simulink model "FMS"  (R2018b)
settings: configuration reference "fms_config" (kept outside this file)
undefined symbols (not defined in the file): actuator_cmd, ay_cmd, ControlMode, ctrl_mode, DiscIntNeverNeededParam, FMS_Cmd, FMS_CONST, FMS_EXPORT, FMS_PARAM, home, mode, p_cmd, phi_cmd, PilotMode, psi_rate_cmd, q_cmd, r_cmd, reset, state, status, theta_cmd, throttle_cmd, timestamp, u_cmd, v_cmd, VehicleState, VehicleStatus, w_cmd, wp_consume, wp_current
libraries: FMT_Model_Lib x41, simulink x27
(part 2 of 4)

== system FMS/FMS_Commander/Commander/Arm/Assist/Altitude/Heading Command ==
  FMS_In : Inport
  Bus Selector : BusSelector  OutputSignals=Pilot_Cmd.stick_yaw
  DeadZone : Subsystem  mask{th=FMS_PARAM.YAW_DZ}
      mask prompts: th "Threshold"
      mask Display: disp('Dead Zone')
  Gain1 : Gain  Gain=FMS_PARAM.YAW_RATE_LIM  OutDataTypeStr=single
  TD : Subsystem
  psi_rate_cmd_radPs : Outport  VectorParamsAs1DForOutWhenUnconnected=off
  wires:
  FMS_In/1 -> Bus Selector/1
  DeadZone/1(y) -> Gain1/1
  Bus Selector/1 -> DeadZone/1(u)  "<stick_yaw>"
  Gain1/1 -> TD/1(v)
  TD/1(v1) -> psi_rate_cmd_radPs/1

== system FMS/FMS_Commander/Commander/Arm/Assist/Position/Airspeed Command ==
  FMS_In : Inport
  Bias : Bias  Bias=1
  Bus Selector : BusSelector  OutputSignals=Pilot_Cmd.stick_throttle
  Gain : Gain  Gain=FMS_PARAM.FW_AIRSPD_MAX
  Gain1 : Gain  Gain=0.5
  Saturation : Saturate  UpperLimit=1  LowerLimit=0
  u_cmd_mPs : Outport  VectorParamsAs1DForOutWhenUnconnected=off
  wires:
  FMS_In/1 -> Bus Selector/1
  Gain/1 -> u_cmd_mPs/1
  Bus Selector/1 -> Bias/1  "<stick_throttle>"
  Bias/1 -> Gain1/1
  Gain1/1 -> Saturation/1
  Saturation/1 -> Gain/1

== system FMS/FMS_Commander/Commander/Arm/Assist/Position/Altitude Command ==
  FMS_In : Inport
  Controller : Subsystem
  Detect Movement : Subsystem
  w_cmd_mPs : Outport  VectorParamsAs1DForOutWhenUnconnected=off
  wires:
  Controller/1(w_cmd_mPs) -> w_cmd_mPs/1
  Detect Movement/1(motion_state) -> Controller/1(motion_state)
  FMS_In/1 -> Controller/2(FMS_In), Detect Movement/1(FMS_In)

== system FMS/FMS_Commander/Commander/Arm/Assist/Position/Heading Command ==
  FMS_In : Inport
  Bus Selector : BusSelector  OutputSignals=Pilot_Cmd.stick_yaw
  DeadZone : Subsystem  mask{th=FMS_PARAM.YAW_DZ}
      mask prompts: th "Threshold"
      mask Display: disp('Dead Zone')
  Gain1 : Gain  Gain=FMS_PARAM.YAW_RATE_LIM  OutDataTypeStr=single
  TD : Subsystem
  psi_rate_cmd_radPs : Outport  VectorParamsAs1DForOutWhenUnconnected=off
  wires:
  Gain1/1 -> TD/1(v)
  FMS_In/1 -> Bus Selector/1
  DeadZone/1(y) -> Gain1/1
  Bus Selector/1 -> DeadZone/1(u)  "<stick_yaw>"
  TD/1(v1) -> psi_rate_cmd_radPs/1

== system FMS/FMS_Commander/Commander/Arm/Assist/Position/Position Command ==
  FMS_In : Inport
  Controller : Subsystem
  Detect Movement : Subsystem
  ay_cmd_mPs2 : Outport  VectorParamsAs1DForOutWhenUnconnected=off
  wires:
  FMS_In/1 -> Controller/2(FMS_In), Detect Movement/1(FMS_In)
  Controller/1(ay_cmd_mPs2) -> ay_cmd_mPs2/1
  Detect Movement/1(motion_state) -> Controller/1(motion_state)

== system FMS/FMS_Commander/Commander/Arm/Assist/Stabilize/Attitude Command ==
  FMS_In : Inport
  Bus Selector : BusSelector  OutputSignals=Pilot_Cmd.stick_roll,Pilot_Cmd.stick_pitch
  DeadZone : Subsystem  mask{th=FMS_PARAM.ROLL_DZ}
      mask prompts: th "Threshold"
      mask Display: disp('Dead Zone')
  DeadZone2 : Subsystem  mask{th=FMS_PARAM.PITCH_DZ}
      mask prompts: th "Threshold"
      mask Display: disp('Dead Zone')
  Gain : Gain  Gain=FMS_PARAM.ROLL_LIM
  Gain1 : Gain  Gain=-FMS_PARAM.PITCH_LIM
  Phi_CMD_TD : Subsystem  Commented=on
  Theta_CMD_TD : Subsystem  Commented=on
  phi_cmd_radPs : Outport  VectorParamsAs1DForOutWhenUnconnected=off
  theta_cmd_radPs : Outport  Port=2  VectorParamsAs1DForOutWhenUnconnected=off
  wires:
  Bus Selector/2 -> DeadZone2/1(u)  "<stick_pitch>"
  Bus Selector/1 -> DeadZone/1(u)  "<stick_roll>"
  FMS_In/1 -> Bus Selector/1
  DeadZone2/1(y) -> Gain1/1
  DeadZone/1(y) -> Gain/1
  Gain/1 -> phi_cmd_radPs/1
  Gain1/1 -> theta_cmd_radPs/1

== system FMS/FMS_Commander/Commander/Arm/Assist/Stabilize/Heading Command ==
  FMS_In : Inport
  Bus Selector : BusSelector  OutputSignals=Pilot_Cmd.stick_yaw
  DeadZone : Subsystem  mask{th=FMS_PARAM.YAW_DZ}
      mask prompts: th "Threshold"
      mask Display: disp('Dead Zone')
  Gain1 : Gain  Gain=FMS_PARAM.YAW_RATE_LIM  OutDataTypeStr=single
  TD : Subsystem  Commented=on
  psi_rate_cmd_radPs : Outport  VectorParamsAs1DForOutWhenUnconnected=off
  wires:
  Gain1/1 -> psi_rate_cmd_radPs/1
  FMS_In/1 -> Bus Selector/1
  DeadZone/1(y) -> Gain1/1
  Bus Selector/1 -> DeadZone/1(u)  "<stick_yaw>"

== system FMS/FMS_Commander/Commander/Arm/Assist/Stabilize/Throttle Command ==
  FMS_In : Inport
  Add : Sum
  Bus Selector : BusSelector  OutputSignals=Pilot_Cmd.stick_throttle
  Constant4 : Constant  OutDataTypeStr=single
  Constant5 : Constant  Value=1000  OutDataTypeStr=uint16
  Gain2 : Gain  Gain=500  OutDataTypeStr=uint16
  Saturation : Saturate  UpperLimit=2  LowerLimit=0
  Sum : Sum  Inputs=|++
  throttle_cmd : Outport  VectorParamsAs1DForOutWhenUnconnected=off
  wires:
  FMS_In/1 -> Bus Selector/1
  Gain2/1 -> Add/1
  Sum/1 -> Saturation/1
  Saturation/1 -> Gain2/1
  Bus Selector/1 -> Sum/1  "<stick_throttle>"
  Constant5/1 -> Add/2
  Add/1 -> throttle_cmd/1
  Constant4/1 -> Sum/2

== system FMS/FMS_Commander/Commander/Arm/Auto/Mission/Mission_SubSystem ==
  FMS_In : Inport
  Reset : ResetPort  DisableCoverage=on
  Altitude Control : Subsystem
  Bus Assignment : BusAssignment  AssignedSignals=status,state,ctrl_mode,u_cmd,ay_cmd,w_cmd
  Constant : Constant  Value=0  OutDataTypeStr=Bus: FMS_Out_Bus
  Constant1 : Constant  Value=VehicleStatus.Arm
  Constant2 : Constant  Value=VehicleState.Mission
  Constant3 : Constant  Value=ControlMode.POSCTL
  Cruise Speed : Subsystem
  Data Type Conversion : DataTypeConversion
  Data Type Conversion1 : DataTypeConversion
  Data Type Conversion2 : DataTypeConversion
  Position Command : Subsystem
  FMS_Out : Outport  VectorParamsAs1DForOutWhenUnconnected=off
  wires:
  Data Type Conversion1/1 -> Bus Assignment/3
  Constant1/1 -> Data Type Conversion/1
  Data Type Conversion2/1 -> Bus Assignment/4
  Data Type Conversion/1 -> Bus Assignment/2
  Constant2/1 -> Data Type Conversion1/1
  Constant3/1 -> Data Type Conversion2/1
  Constant/1 -> Bus Assignment/1
  Bus Assignment/1 -> FMS_Out/1
  Position Command/1(ay_cmd_mPs2) -> Bus Assignment/6
  Altitude Control/1(w_cmd_mPs) -> Bus Assignment/7
  Cruise Speed/1(cruise_speed) -> Bus Assignment/5
  FMS_In/1 -> Cruise Speed/1(FMS_In), Altitude Control/1(FMS_In), Position Command/1(FMS_In)

== system FMS/FMS_Commander/Commander/Arm/Manual/Manual_Cmd/throttle ==
  stick_throttle : Inport
  Add : Sum
  Constant4 : Constant  OutDataTypeStr=single
  Constant5 : Constant  Value=1000  OutDataTypeStr=single
  Gain4 : Gain  Gain=500  OutDataTypeStr=Inherit: Same as input
  Saturation : Saturate  UpperLimit=2  LowerLimit=0
  Sum : Sum  Inputs=|++
  throttle_cmd : Outport  VectorParamsAs1DForOutWhenUnconnected=off
  wires:
  stick_throttle/1 -> Sum/1
  Sum/1 -> Saturation/1
  Constant4/1 -> Sum/2
  Saturation/1 -> Gain4/1
  Add/1 -> throttle_cmd/1
  Gain4/1 -> Add/1
  Constant5/1 -> Add/2

== system FMS/FMS_Commander/Commander/Arm/SubMode/Hold/Altitude_Hold ==
  FMS_In : Inport
  Bus_Selection : Subsystem
  Delay : Delay  DelayLength=1  InitialConditionSource=Input port
      settings: InputPortMap=u0,p4
  Gain2 : Gain  Gain=FMS_PARAM.Z_P  OutDataTypeStr=single
  Saturation1 : Saturate  UpperLimit=FMS_PARAM.VEL_Z_LIM  LowerLimit=-FMS_PARAM.VEL_Z_LIM
  Sum : Sum  Inputs=-+|
  w_cmd_mPs : Outport  VectorParamsAs1DForOutWhenUnconnected=off
  wires:
  Gain2/1 -> Saturation1/1
  Bus_Selection/1(z_R_m) -> Delay/2, Sum/1  "z_est_R"
  Sum/1 -> Gain2/1  "z_err_R"
  Delay/1 -> Sum/2, Delay/1  "z_cmd_R"
  FMS_In/1 -> Bus_Selection/1(FMS_In)
  Saturation1/1 -> w_cmd_mPs/1

== system FMS/FMS_Commander/Commander/Arm/SubMode/Hold/Loiter_Control ==
  FMS_In : Inport
  Bus Selector2 : BusSelector  OutputSignals=INS_Out.vn,INS_Out.ve
  L1 : Constant  Value=FMS_PARAM.L1  OutDataTypeStr=single
  L1 Reference WP : Subsystem
  L1_Core : Subsystem
  Mux1 : Mux  Inputs=2
  R : Constant  Value=FMS_PARAM.LOITER_R  OutDataTypeStr=single
  Reference_Point : Subsystem
  ay_cmd_mPs2 : Outport  VectorParamsAs1DForOutWhenUnconnected=off
  wires:
  L1 Reference WP/1(L1_WP) -> L1_Core/2(L1_WP)  "L1_WP"
  L1_Core/1(ay_cmd_mPs2) -> ay_cmd_mPs2/1
  Reference_Point/1(p_vehicle) -> L1_Core/1(p_vehicle), L1 Reference WP/1(P_Vehicle)
  Reference_Point/2(p_0) -> L1 Reference WP/2(P_0)
  Reference_Point/3(n) -> L1 Reference WP/3(n)
  R/1 -> L1 Reference WP/4(R)
  L1/1 -> L1_Core/3(L1), L1 Reference WP/5(L1)
  FMS_In/1 -> Bus Selector2/1, Reference_Point/1(FMS_In)
  Bus Selector2/2 -> Mux1/2  "<ve>"
  Bus Selector2/1 -> Mux1/1  "<vn>"
  Mux1/1 -> L1_Core/4(Vg)

== system FMS/FMS_Commander/Commander/Arm/SubMode/Return/Altitude Control ==
  FMS_In : Inport
  Bus Selector3 : BusSelector  OutputSignals=INS_Out.h_R
  Gain : Gain  Gain=FMS_PARAM.Z_P
  Saturation1 : Saturate  UpperLimit=FMS_PARAM.VEL_Z_LIM  LowerLimit=-FMS_PARAM.VEL_Z_LIM
  Sum2 : Sum  Inputs=|+-
  Target Height : Subsystem
  w_cmd_mPs : Outport  VectorParamsAs1DForOutWhenUnconnected=off
  wires:
  FMS_In/1 -> Bus Selector3/1, Target Height/1(FMS_In)
  Bus Selector3/1 -> Sum2/1  "<h_R>"
  Sum2/1 -> Gain/1
  Gain/1 -> Saturation1/1
  Target Height/1(h_R_sp) -> Sum2/2  "h_R_sp"
  Saturation1/1 -> w_cmd_mPs/1

== system FMS/FMS_Commander/Commander/Arm/SubMode/Return/Cruise Speed ==
  FMS_In : Inport
  Bus Selector : BusSelector  OutputSignals=Cmd_In.set_speed
  Compare To Zero : simulink/Logic and Bit Operations/Compare To Zero  relop=>  OutDataTypeStr=boolean
  Switch2 : Switch  Criteria=u2 > Threshold
  vel : Constant  Value=FMS_PARAM.CRUISE_SPEED  OutDataTypeStr=single
  cruise_speed : Outport  VectorParamsAs1DForOutWhenUnconnected=off
  wires:
  Bus Selector/1 -> Compare To Zero/1, Switch2/1  "<set_speed>"
  vel/1 -> Switch2/3  "|Vg|"
  Compare To Zero/1 -> Switch2/2
  Switch2/1 -> cruise_speed/1
  FMS_In/1 -> Bus Selector/1

== system FMS/FMS_Commander/Commander/Arm/SubMode/Return/Position Command ==
  FMS_In : Inport
  L1 Control : Subsystem
  WayPoints : Subsystem
  ay_cmd_mPs2 : Outport  VectorParamsAs1DForOutWhenUnconnected=off
  wires:
  FMS_In/1 -> L1 Control/4(FMS_In), WayPoints/1(FMS_In)
  L1 Control/1(ay_cmd_mPs2) -> ay_cmd_mPs2/1
  WayPoints/2(p2) -> L1 Control/2(p2)
  WayPoints/3(p3) -> L1 Control/3(p3)
  WayPoints/1(p1) -> L1 Control/1(p1)

== system FMS/FMS_Commander/Commander/Arm/SubMode/Takeoff/Altitude Control ==
  FMS_In : Inport
  Bus Selector3 : BusSelector  OutputSignals=INS_Out.h_R
  Gain : Gain  Gain=FMS_PARAM.Z_P
  Saturation1 : Saturate  UpperLimit=FMS_PARAM.VEL_Z_LIM  LowerLimit=-FMS_PARAM.VEL_Z_LIM
  Sum2 : Sum  Inputs=|+-
  Target Height : Subsystem
  w_cmd_mPs : Outport  VectorParamsAs1DForOutWhenUnconnected=off
  wires:
  FMS_In/1 -> Bus Selector3/1, Target Height/1(FMS_In)
  Bus Selector3/1 -> Sum2/1  "<h_R>"
  Sum2/1 -> Gain/1
  Gain/1 -> Saturation1/1
  Target Height/1(h_R_sp) -> Sum2/2  "h_R_sp"
  Saturation1/1 -> w_cmd_mPs/1

== system FMS/FMS_Commander/Commander/Arm/SubMode/Takeoff/Position Command ==
  FMS_In : Inport
  L1 Control : Subsystem
  WayPoints : Subsystem
  ay_cmd_mPs2 : Outport  VectorParamsAs1DForOutWhenUnconnected=off
  wires:
  FMS_In/1 -> L1 Control/4(FMS_In), WayPoints/1(FMS_In)
  L1 Control/1(ay_cmd_mPs2) -> ay_cmd_mPs2/1
  WayPoints/2(p2) -> L1 Control/2(p2)
  WayPoints/3(p3) -> L1 Control/3(p3)
  WayPoints/1(p1) -> L1 Control/1(p1)

== system FMS/FMS_Commander/Commander/Arm/Assist/Altitude/Airspeed Command/TD ==
  v : Inport
  Integrator : DiscreteIntegrator  SampleTime=-1  ICPrevOutput=DiscIntNeverNeededParam  ICPrevScaledInput=DiscIntNeverNeededParam
  Integrator1 : DiscreteIntegrator  SampleTime=-1  ICPrevOutput=DiscIntNeverNeededParam  ICPrevScaledInput=DiscIntNeverNeededParam
  Subtract : Sum  Inputs=+-
  "fhan " : Subsystem  mask{r0=8*9.806, h0=0.05}
      mask DialogControl ParameterGroupVar Prompt: fhan(v1,v2,r0,h0)
  v1 : Outport  VectorParamsAs1DForOutWhenUnconnected=off
  wires:
  Integrator1/1 -> v1/1, Subtract/1
  v/1 -> Subtract/2
  Integrator/1 -> "fhan "/2(v2), Integrator1/1  "v2"
  Subtract/1 -> "fhan "/1(v1)
  "fhan "/1(fhan) -> Integrator/1

== system FMS/FMS_Commander/Commander/Arm/Assist/Altitude/Altitude Command/Controller ==
  motion_state : Inport
  In Bus Element : Inport  Port=2  PortName=FMS_In
  In Bus Element1 : Inport  Port=2  PortName=FMS_In
  Brake Control : Subsystem  TreatAsAtomicUnit=on
  Hold Control : Subsystem  TreatAsAtomicUnit=on
  Merge : Merge  Inputs=3
  Move Control : Subsystem  TreatAsAtomicUnit=on
  Saturation1 : Saturate  UpperLimit=FMS_PARAM.VEL_Z_LIM  LowerLimit=-FMS_PARAM.VEL_Z_LIM
  Switch Case : SwitchCase  CaseConditions={MotionState.Hold, MotionState.Brake, MotionState.Move}  ShowDefaultCase=off
  w_cmd_mPs : Outport  VectorParamsAs1DForOutWhenUnconnected=off
  wires:
  Move Control/1(w_cmd_mPs) -> Merge/3
  Brake Control/1(psi_rate_cmd_radPs) -> Merge/2
  Hold Control/1(w_cmd_mPs) -> Merge/1
  In Bus Element/1 -> Hold Control/1(FMS_In)
  Switch Case/3 -> Move Control/Action
  Switch Case/2 -> Brake Control/Action
  Switch Case/1 -> Hold Control/Action
  motion_state/1 -> Switch Case/1
  Saturation1/1 -> w_cmd_mPs/1
  Merge/1 -> Saturation1/1
  In Bus Element1/1 -> Move Control/1(FMS_In)

== system FMS/FMS_Commander/Commander/Arm/Assist/Altitude/Altitude Command/Detect Movement ==
  FMS_In : Inport
  Abs : Abs
  Abs1 : Abs
  Bus Selector : BusSelector  OutputSignals=Pilot_Cmd.stick_pitch,INS_Out.vd
  Compare To Constant : simulink/Logic and Bit Operations/Compare To Constant  relop=>  const=FMS_PARAM.PITCH_DZ  OutDataTypeStr=boolean
  Motion Status : Stateflow chart  TreatAsAtomicUnit=on
  motion_state : Outport  VectorParamsAs1DForOutWhenUnconnected=off
  wires:
  FMS_In/1 -> Bus Selector/1
  Abs1/1 -> Compare To Constant/1
  Motion Status/1(state) -> motion_state/1
  Compare To Constant/1 -> Motion Status/1(motion_req)
  Abs/1 -> Motion Status/2(speed)
  Bus Selector/1 -> Abs1/1  "<stick_pitch>"
  Bus Selector/2 -> Abs/1  "<vd>"

== system FMS/FMS_Commander/Commander/Arm/Assist/Altitude/Attitude Command/DeadZone ==
  u : Inport
  Dead Zone : DeadZone  LowerValue=-th  UpperValue=th  SaturateOnIntegerOverflow=on
  Gain : Gain  Gain=1/(1-th)
  y : Outport  VectorParamsAs1DForOutWhenUnconnected=off
  wires:
  Gain/1 -> y/1
  Dead Zone/1 -> Gain/1
  u/1 -> Dead Zone/1

== system FMS/FMS_Commander/Commander/Arm/Assist/Altitude/Attitude Command/Phi_CMD_TD ==
  v : Inport
  Integrator : DiscreteIntegrator  SampleTime=-1  ICPrevOutput=DiscIntNeverNeededParam  ICPrevScaledInput=DiscIntNeverNeededParam
  Integrator1 : DiscreteIntegrator  SampleTime=-1  ICPrevOutput=DiscIntNeverNeededParam  ICPrevScaledInput=DiscIntNeverNeededParam
  Subtract : Sum  Inputs=+-
  "fhan " : Subsystem  mask{r0=4*pi, h0=0.04}
      mask DialogControl ParameterGroupVar Prompt: fhan(v1,v2,r0,h0)
  v1 : Outport  VectorParamsAs1DForOutWhenUnconnected=off
  wires:
  "fhan "/1(fhan) -> Integrator/1
  Subtract/1 -> "fhan "/1(v1)
  Integrator/1 -> Integrator1/1, "fhan "/2(v2)  "v2"
  v/1 -> Subtract/2
  Integrator1/1 -> Subtract/1, v1/1

== system FMS/FMS_Commander/Commander/Arm/Assist/Altitude/Heading Command/DeadZone ==
  u : Inport
  Dead Zone : DeadZone  LowerValue=-th  UpperValue=th  SaturateOnIntegerOverflow=on
  Gain : Gain  Gain=1/(1-th)
  y : Outport  VectorParamsAs1DForOutWhenUnconnected=off
  wires:
  Gain/1 -> y/1
  Dead Zone/1 -> Gain/1
  u/1 -> Dead Zone/1

== system FMS/FMS_Commander/Commander/Arm/Assist/Altitude/Heading Command/TD ==
  v : Inport
  Integrator : DiscreteIntegrator  SampleTime=-1  ICPrevOutput=DiscIntNeverNeededParam  ICPrevScaledInput=DiscIntNeverNeededParam
  Integrator1 : DiscreteIntegrator  SampleTime=-1  ICPrevOutput=DiscIntNeverNeededParam  ICPrevScaledInput=DiscIntNeverNeededParam
  Subtract : Sum  Inputs=+-
  "fhan " : Subsystem  mask{r0=5*pi, h0=0.02}
      mask DialogControl ParameterGroupVar Prompt: fhan(v1,v2,r0,h0)
  v1 : Outport  VectorParamsAs1DForOutWhenUnconnected=off
  wires:
  "fhan "/1(fhan) -> Integrator/1
  Subtract/1 -> "fhan "/1(v1)
  Integrator/1 -> Integrator1/1, "fhan "/2(v2)  "v2"
  v/1 -> Subtract/2
  Integrator1/1 -> Subtract/1, v1/1

== system FMS/FMS_Commander/Commander/Arm/Assist/Position/Altitude Command/Controller ==
  motion_state : Inport
  In Bus Element : Inport  Port=2  PortName=FMS_In
  In Bus Element1 : Inport  Port=2  PortName=FMS_In
  Brake Control : Subsystem  TreatAsAtomicUnit=on
  Hold Control : Subsystem  TreatAsAtomicUnit=on
  Merge : Merge  Inputs=3
  Move Control : Subsystem  TreatAsAtomicUnit=on
  Saturation1 : Saturate  UpperLimit=FMS_PARAM.VEL_Z_LIM  LowerLimit=-FMS_PARAM.VEL_Z_LIM
  Switch Case : SwitchCase  CaseConditions={MotionState.Hold, MotionState.Brake, MotionState.Move}  ShowDefaultCase=off
  w_cmd_mPs : Outport  VectorParamsAs1DForOutWhenUnconnected=off
  wires:
  Move Control/1(w_cmd_mPs) -> Merge/3
  Brake Control/1(psi_rate_cmd_radPs) -> Merge/2
  Hold Control/1(w_cmd_mPs) -> Merge/1
  In Bus Element/1 -> Hold Control/1(FMS_In)
  Switch Case/3 -> Move Control/Action
  Switch Case/2 -> Brake Control/Action
  Switch Case/1 -> Hold Control/Action
  motion_state/1 -> Switch Case/1
  Saturation1/1 -> w_cmd_mPs/1
  Merge/1 -> Saturation1/1
  In Bus Element1/1 -> Move Control/1(FMS_In)

== system FMS/FMS_Commander/Commander/Arm/Assist/Position/Altitude Command/Detect Movement ==
  FMS_In : Inport
  Abs : Abs
  Abs1 : Abs
  Bus Selector : BusSelector  OutputSignals=Pilot_Cmd.stick_pitch,INS_Out.vd
  Compare To Constant : simulink/Logic and Bit Operations/Compare To Constant  relop=>  const=FMS_PARAM.PITCH_DZ  OutDataTypeStr=boolean
  Motion Status : Stateflow chart  TreatAsAtomicUnit=on
  motion_state : Outport  VectorParamsAs1DForOutWhenUnconnected=off
  wires:
  FMS_In/1 -> Bus Selector/1
  Abs1/1 -> Compare To Constant/1
  Motion Status/1(state) -> motion_state/1
  Compare To Constant/1 -> Motion Status/1(motion_req)
  Abs/1 -> Motion Status/2(speed)
  Bus Selector/1 -> Abs1/1  "<stick_pitch>"
  Bus Selector/2 -> Abs/1  "<vd>"

== system FMS/FMS_Commander/Commander/Arm/Assist/Position/Heading Command/DeadZone ==
  u : Inport
  Dead Zone : DeadZone  LowerValue=-th  UpperValue=th  SaturateOnIntegerOverflow=on
  Gain : Gain  Gain=1/(1-th)
  y : Outport  VectorParamsAs1DForOutWhenUnconnected=off
  wires:
  Gain/1 -> y/1
  Dead Zone/1 -> Gain/1
  u/1 -> Dead Zone/1

== system FMS/FMS_Commander/Commander/Arm/Assist/Position/Heading Command/TD ==
  v : Inport
  Integrator : DiscreteIntegrator  SampleTime=-1  ICPrevOutput=DiscIntNeverNeededParam  ICPrevScaledInput=DiscIntNeverNeededParam
  Integrator1 : DiscreteIntegrator  SampleTime=-1  ICPrevOutput=DiscIntNeverNeededParam  ICPrevScaledInput=DiscIntNeverNeededParam
  Subtract : Sum  Inputs=+-
  "fhan " : Subsystem  mask{r0=5*pi, h0=0.02}
      mask DialogControl ParameterGroupVar Prompt: fhan(v1,v2,r0,h0)
  v1 : Outport  VectorParamsAs1DForOutWhenUnconnected=off
  wires:
  "fhan "/1(fhan) -> Integrator/1
  Subtract/1 -> "fhan "/1(v1)
  Integrator/1 -> Integrator1/1, "fhan "/2(v2)  "v2"
  v/1 -> Subtract/2
  Integrator1/1 -> Subtract/1, v1/1

== system FMS/FMS_Commander/Commander/Arm/Assist/Position/Position Command/Controller ==
  motion_state : Inport
  In Bus Element : Inport  Port=2  PortName=FMS_In
  In Bus Element1 : Inport  Port=2  PortName=FMS_In
  Brake Control : Subsystem  TreatAsAtomicUnit=on
  Hold Control : Subsystem  TreatAsAtomicUnit=on
  Merge : Merge  Inputs=3
  Move Control : Subsystem  TreatAsAtomicUnit=on
  Saturation1 : Saturate  UpperLimit=FMS_PARAM.ACC_Y_LIM  LowerLimit=-FMS_PARAM.ACC_Y_LIM
  Switch Case : SwitchCase  CaseConditions={MotionState.Hold, MotionState.Brake, MotionState.Move}  ShowDefaultCase=off
  ay_cmd_mPs2 : Outport  VectorParamsAs1DForOutWhenUnconnected=off
  wires:
  Move Control/1(ay_cmd_mPs2) -> Merge/3
  Brake Control/1(ay_cmd_mPs2) -> Merge/2
  Hold Control/1(ay_cmd_mPs2) -> Merge/1
  In Bus Element/1 -> Hold Control/1(FMS_In)
  Switch Case/3 -> Move Control/Action
  Switch Case/2 -> Brake Control/Action
  Switch Case/1 -> Hold Control/Action
  motion_state/1 -> Switch Case/1
  Saturation1/1 -> ay_cmd_mPs2/1
  Merge/1 -> Saturation1/1
  In Bus Element1/1 -> Move Control/1(FMS_In)

== system FMS/FMS_Commander/Commander/Arm/Assist/Position/Position Command/Detect Movement ==
  FMS_In : Inport
  Abs : Abs
  Abs1 : Abs
  Bus Selector1 : BusSelector  OutputSignals=Pilot_Cmd.stick_roll
  Bus Selector2 : BusSelector  OutputSignals=INS_Out.psi,INS_Out.vn,INS_Out.ve,INS_Out.vd
  Compare To Constant : simulink/Logic and Bit Operations/Compare To Constant  relop=>  const=FMS_PARAM.ROLL_DZ  OutDataTypeStr=boolean
  Motion State : Stateflow chart  TreatAsAtomicUnit=on
  Multiply : Product  Multiplication=Matrix(*)
  Mux : Mux  Inputs=3
  Psi To DCM : FMT_Model_Lib/Transformation/Psi To DCM
      settings: SourceProductName=FMT Toolbox
  Selector : Selector  InputPortWidth=3  IndexOptions=Index vector (dialog)  Indices=2  OutputSizes=1
  motion_state : Outport  VectorParamsAs1DForOutWhenUnconnected=off
  wires:
  FMS_In/1 -> Bus Selector2/1, Bus Selector1/1
  Compare To Constant/1 -> Motion State/1(motion_req)
  Abs1/1 -> Compare To Constant/1
  Motion State/1(state) -> motion_state/1  "pos_ms"
  Abs/1 -> Motion State/2(speed)
  Bus Selector1/1 -> Abs1/1  "<stick_roll>"
  Bus Selector2/1 -> Psi To DCM/1  "<psi>"
  Bus Selector2/2 -> Mux/1  "<vn>"
  Bus Selector2/3 -> Mux/2  "<ve>"
  Bus Selector2/4 -> Mux/3  "<vd>"
  Psi To DCM/1 -> Multiply/1
  Multiply/1 -> Selector/1
  Selector/1 -> Abs/1
  Mux/1 -> Multiply/2

== system FMS/FMS_Commander/Commander/Arm/Assist/Stabilize/Attitude Command/DeadZone ==
  u : Inport
  Dead Zone : DeadZone  LowerValue=-th  UpperValue=th  SaturateOnIntegerOverflow=on
  Gain : Gain  Gain=1/(1-th)
  y : Outport  VectorParamsAs1DForOutWhenUnconnected=off
  wires:
  Gain/1 -> y/1
  Dead Zone/1 -> Gain/1
  u/1 -> Dead Zone/1

== system FMS/FMS_Commander/Commander/Arm/Assist/Stabilize/Attitude Command/DeadZone2 ==
  u : Inport
  Dead Zone : DeadZone  LowerValue=-th  UpperValue=th  SaturateOnIntegerOverflow=on
  Gain : Gain  Gain=1/(1-th)
  y : Outport  VectorParamsAs1DForOutWhenUnconnected=off
  wires:
  u/1 -> Dead Zone/1
  Dead Zone/1 -> Gain/1
  Gain/1 -> y/1

== system FMS/FMS_Commander/Commander/Arm/Assist/Stabilize/Attitude Command/Phi_CMD_TD ==
  v : Inport
  Integrator : DiscreteIntegrator  SampleTime=-1  ICPrevOutput=DiscIntNeverNeededParam  ICPrevScaledInput=DiscIntNeverNeededParam
  Integrator1 : DiscreteIntegrator  SampleTime=-1  ICPrevOutput=DiscIntNeverNeededParam  ICPrevScaledInput=DiscIntNeverNeededParam
  Subtract : Sum  Inputs=+-
  "fhan " : Subsystem  mask{r0=4*pi, h0=0.04}
      mask DialogControl ParameterGroupVar Prompt: fhan(v1,v2,r0,h0)
  v1 : Outport  VectorParamsAs1DForOutWhenUnconnected=off
  wires:
  "fhan "/1(fhan) -> Integrator/1
  Subtract/1 -> "fhan "/1(v1)
  Integrator/1 -> Integrator1/1, "fhan "/2(v2)  "v2"
  v/1 -> Subtract/2
  Integrator1/1 -> Subtract/1, v1/1

== system FMS/FMS_Commander/Commander/Arm/Assist/Stabilize/Attitude Command/Theta_CMD_TD ==
  v : Inport
  Integrator : DiscreteIntegrator  SampleTime=-1  ICPrevOutput=DiscIntNeverNeededParam  ICPrevScaledInput=DiscIntNeverNeededParam
  Integrator1 : DiscreteIntegrator  SampleTime=-1  ICPrevOutput=DiscIntNeverNeededParam  ICPrevScaledInput=DiscIntNeverNeededParam
  Subtract : Sum  Inputs=+-
  "fhan " : Subsystem  mask{r0=4*pi, h0=0.04}
      mask DialogControl ParameterGroupVar Prompt: fhan(v1,v2,r0,h0)
  v1 : Outport  VectorParamsAs1DForOutWhenUnconnected=off
  wires:
  Integrator1/1 -> v1/1, Subtract/1
  v/1 -> Subtract/2
  Integrator/1 -> Integrator1/1, "fhan "/2(v2)  "v2"
  Subtract/1 -> "fhan "/1(v1)
  "fhan "/1(fhan) -> Integrator/1

== system FMS/FMS_Commander/Commander/Arm/Assist/Stabilize/Heading Command/DeadZone ==
  u : Inport
  Dead Zone : DeadZone  LowerValue=-th  UpperValue=th  SaturateOnIntegerOverflow=on
  Gain : Gain  Gain=1/(1-th)
  y : Outport  VectorParamsAs1DForOutWhenUnconnected=off
  wires:
  Gain/1 -> y/1
  Dead Zone/1 -> Gain/1
  u/1 -> Dead Zone/1

== system FMS/FMS_Commander/Commander/Arm/Assist/Stabilize/Heading Command/TD ==
  v : Inport
  Integrator : DiscreteIntegrator  SampleTime=-1  ICPrevOutput=DiscIntNeverNeededParam  ICPrevScaledInput=DiscIntNeverNeededParam
  Integrator1 : DiscreteIntegrator  SampleTime=-1  ICPrevOutput=DiscIntNeverNeededParam  ICPrevScaledInput=DiscIntNeverNeededParam
  Subtract : Sum  Inputs=+-
  "fhan " : Subsystem  mask{r0=5*pi, h0=0.02}
      mask DialogControl ParameterGroupVar Prompt: fhan(v1,v2,r0,h0)
  v1 : Outport  VectorParamsAs1DForOutWhenUnconnected=off
  wires:
  "fhan "/1(fhan) -> Integrator/1
  Subtract/1 -> "fhan "/1(v1)
  Integrator/1 -> Integrator1/1, "fhan "/2(v2)  "v2"
  v/1 -> Subtract/2
  Integrator1/1 -> Subtract/1, v1/1

== system FMS/FMS_Commander/Commander/Arm/Auto/Mission/Mission_SubSystem/Altitude Control ==
  FMS_In : Inport
  Bus Selector3 : BusSelector  OutputSignals=INS_Out.h_R
  Gain : Gain  Gain=FMS_PARAM.Z_P
  Saturation1 : Saturate  UpperLimit=FMS_PARAM.VEL_Z_LIM  LowerLimit=-FMS_PARAM.VEL_Z_LIM
  Sum2 : Sum  Inputs=|+-
  Target Height : Subsystem
  w_cmd_mPs : Outport  VectorParamsAs1DForOutWhenUnconnected=off
  wires:
  FMS_In/1 -> Bus Selector3/1, Target Height/1(FMS_In)
  Bus Selector3/1 -> Sum2/1  "<h_R>"
  Sum2/1 -> Gain/1
  Gain/1 -> Saturation1/1
  Target Height/1(h_R_sp) -> Sum2/2  "h_R_sp"
  Saturation1/1 -> w_cmd_mPs/1

== system FMS/FMS_Commander/Commander/Arm/Auto/Mission/Mission_SubSystem/Cruise Speed ==
  FMS_In : Inport
  Bus Selector : BusSelector  OutputSignals=Cmd_In.set_speed
  Compare To Zero : simulink/Logic and Bit Operations/Compare To Zero  relop=>  OutDataTypeStr=boolean
  Switch2 : Switch  Criteria=u2 > Threshold
  vel : Constant  Value=FMS_PARAM.CRUISE_SPEED  OutDataTypeStr=single
  cruise_speed : Outport  VectorParamsAs1DForOutWhenUnconnected=off
  wires:
  Bus Selector/1 -> Compare To Zero/1, Switch2/1  "<set_speed>"
  vel/1 -> Switch2/3  "|Vg|"
  Compare To Zero/1 -> Switch2/2
  Switch2/1 -> cruise_speed/1
  FMS_In/1 -> Bus Selector/1

== system FMS/FMS_Commander/Commander/Arm/Auto/Mission/Mission_SubSystem/Position Command ==
  FMS_In : Inport
  L1 Control : Subsystem
  WayPoints : Subsystem
  ay_cmd_mPs2 : Outport  VectorParamsAs1DForOutWhenUnconnected=off
  wires:
  FMS_In/1 -> L1 Control/4(FMS_In), WayPoints/1(FMS_In)
  L1 Control/1(ay_cmd_mPs2) -> ay_cmd_mPs2/1
  WayPoints/2(p2) -> L1 Control/2(p2)
  WayPoints/3(p3) -> L1 Control/3(p3)
  WayPoints/1(p1) -> L1 Control/1(p1)

== system FMS/FMS_Commander/Commander/Arm/SubMode/Hold/Altitude_Hold/Bus_Selection ==
  FMS_In : Inport
  Bus Selector2 : BusSelector  OutputSignals=INS_Out.h_R
  Gain : Gain  Gain=-1
  z_R_m : Outport  VectorParamsAs1DForOutWhenUnconnected=off
  wires:
  Gain/1 -> z_R_m/1
  Bus Selector2/1 -> Gain/1  "<h_R>"
  FMS_In/1 -> Bus Selector2/1

== system FMS/FMS_Commander/Commander/Arm/SubMode/Hold/Loiter_Control/L1 Reference WP ==
  P_Vehicle : Inport
  P_0 : Inport  Port=2
  n : Inport  Port=3
  R : Inport  Port=4
  L1 : Inport  Port=5
  Compare To Constant : simulink/Logic and Bit Operations/Compare To Constant  relop=>  const=0  OutDataTypeStr=boolean
  Gain : Gain  Gain=0.5
  Max : MinMax  Function=max  Inputs=2
  OutRegionRegWP : MATLAB Function  TreatAsAtomicUnit=on
  Reshape : Reshape  OutputDimensionality=Customize  OutputDimensions=[2,1]
  Reshape1 : Reshape  OutputDimensionality=Column vector (2-D)
  Reshape2 : Reshape  OutputDimensionality=Column vector (2-D)
  Reshape3 : Reshape  OutputDimensionality=Column vector (2-D)
  SearchL1RefWP : MATLAB Function  TreatAsAtomicUnit=on
  Switch : Switch  Criteria=u2 > Threshold
  L1_WP : Outport  VectorParamsAs1DForOutWhenUnconnected=off
  wires:
  Reshape/1 -> L1_WP/1
  Compare To Constant/1 -> Switch/2
  SearchL1RefWP/2(n) -> Compare To Constant/1
  OutRegionRegWP/1(P) -> Switch/3
  Switch/1 -> Reshape/1
  SearchL1RefWP/1(P) -> Switch/1
  P_0/1 -> Reshape1/1
  P_Vehicle/1 -> Reshape2/1
  Max/1 -> OutRegionRegWP/3(R), SearchL1RefWP/3(R)
  L1/1 -> Gain/1, OutRegionRegWP/4(L1), SearchL1RefWP/4(L1)
  Reshape1/1 -> OutRegionRegWP/1(P0), SearchL1RefWP/1(P_0)
  Reshape2/1 -> OutRegionRegWP/2(P_Vehicle), SearchL1RefWP/2(P_Vehicle)
  n/1 -> Reshape3/1
  Reshape3/1 -> OutRegionRegWP/5(n)
  R/1 -> Max/1
  Gain/1 -> Max/2

== system FMS/FMS_Commander/Commander/Arm/SubMode/Hold/Loiter_Control/L1_Core ==
  p_vehicle : Inport
  L1_WP : Inport  Port=2
  L1 : Inport  Port=3
  Vg : Inport  Port=4
  L1_Lateral_Acceleration : Subsystem
  Saturation : Saturate  UpperLimit=9.81  LowerLimit=-9.81
  Subtract : Sum  Inputs=+-
  ay_cmd_mPs2 : Outport  VectorParamsAs1DForOutWhenUnconnected=off
  wires:
  L1_WP/1 -> Subtract/1
  p_vehicle/1 -> Subtract/2
  L1/1 -> L1_Lateral_Acceleration/1(L1)
  Vg/1 -> L1_Lateral_Acceleration/2(Vg)
  Subtract/1 -> L1_Lateral_Acceleration/3(l1_path)
  L1_Lateral_Acceleration/1(l1_a_cmd) -> Saturation/1
  Saturation/1 -> ay_cmd_mPs2/1

== system FMS/FMS_Commander/Commander/Arm/SubMode/Hold/Loiter_Control/Reference_Point ==
  FMS_In : Inport
  Bus Selector1 : BusSelector  OutputSignals=Cmd_In.cur_waypoint
  Bus Selector2 : BusSelector  OutputSignals=INS_Out.vn,INS_Out.ve
  Bus Selector3 : BusSelector  OutputSignals=INS_Out.x_R,INS_Out.y_R
  Mux1 : Mux  Inputs=2
  Mux2 : Mux  Inputs=2
  Selector : Selector  InputPortWidth=3  IndexOptions=Index vector (dialog)  Indices=[1 2]  OutputSizes=1
  Vector Normalize : FMT_Model_Lib/Math/Vector Normalize
      settings: SourceProductName=FMT Toolbox
  start_vel : Delay  DelayLength=1  InitialConditionSource=Input port
      settings: InputPortMap=u0,p4
  p_vehicle : Outport  VectorParamsAs1DForOutWhenUnconnected=off
  p_0 : Outport  Port=2  VectorParamsAs1DForOutWhenUnconnected=off
  n : Outport  Port=3  VectorParamsAs1DForOutWhenUnconnected=off
  wires:
  Bus Selector2/2 -> Mux1/2  "<ve>"
  start_vel/1 -> Vector Normalize/1, start_vel/1
  Bus Selector2/1 -> Mux1/1  "<vn>"
  Vector Normalize/1 -> n/1
  FMS_In/1 -> Bus Selector3/1, Bus Selector2/1, Bus Selector1/1
  Mux1/1 -> start_vel/2
  Bus Selector3/1 -> Mux2/1  "<x_R>"
  Bus Selector3/2 -> Mux2/2  "<y_R>"
  Mux2/1 -> p_vehicle/1
  Bus Selector1/1 -> Selector/1  "<cur_waypoint>"
  Selector/1 -> p_0/1

== system FMS/FMS_Commander/Commander/Arm/SubMode/Return/Altitude Control/Target Height ==
  FMS_In : Inport
  Add : Sum
  Bus Selector : BusSelector  OutputSignals=Cmd_In.sp_waypoint,Cmd_In.cur_waypoint
  Bus Selector1 : BusSelector  OutputSignals=INS_Out.x_R,INS_Out.y_R
  Bus Selector2 : BusSelector  OutputSignals=Cmd_In.cur_waypoint,Cmd_In.sp_waypoint
  Divide : Product  Inputs=*/
  Multiply : Product
  Mux : Mux  Inputs=2
  Saturation : Saturate  UpperLimit=1  LowerLimit=0
  Selector : Selector  InputPortWidth=3  IndexOptions=Index vector (dialog)  Indices=3  OutputSizes=1
  Selector1 : Selector  InputPortWidth=3  IndexOptions=Index vector (dialog)  Indices=3  OutputSizes=1
  Selector2 : Selector  InputPortWidth=3  IndexOptions=Index vector (dialog)  Indices=[1 2]  OutputSizes=1
  Selector3 : Selector  InputPortWidth=3  IndexOptions=Index vector (dialog)  Indices=[1 2]  OutputSizes=1
  Subtract : Sum  Inputs=+-
  Sum : Sum  Inputs=|+-
  Sum1 : Sum  Inputs=-+|
  Vector Modulus : FMT_Model_Lib/Math/Vector Modulus
      settings: SourceProductName=FMT Toolbox
  Vector Modulus1 : FMT_Model_Lib/Math/Vector Modulus
      settings: SourceProductName=FMT Toolbox
  h_R_sp : Outport  VectorParamsAs1DForOutWhenUnconnected=off
  wires:
  Multiply/1 -> Add/2
  Bus Selector1/1 -> Mux/1  "<x_R>"
  Bus Selector/1 -> Selector1/1  "<sp_waypoint>"
  Vector Modulus1/1 -> Divide/2
  Sum1/1 -> Vector Modulus1/1
  Sum/1 -> Vector Modulus/1
  Selector2/1 -> Sum1/1, Sum/2
  FMS_In/1 -> Bus Selector2/1, Bus Selector1/1, Bus Selector/1
  Bus Selector2/2 -> Selector3/1  "<sp_waypoint>"
  Vector Modulus/1 -> Divide/1
  Bus Selector1/2 -> Mux/2  "<y_R>"
  Bus Selector2/1 -> Selector2/1  "<cur_waypoint>"
  Selector1/1 -> Subtract/1
  Mux/1 -> Sum/1
  Subtract/1 -> Multiply/1
  Divide/1 -> Saturation/1
  Selector3/1 -> Sum1/2
  Bus Selector/2 -> Selector/1  "<cur_waypoint>"
  Selector/1 -> Add/1, Subtract/2
  Saturation/1 -> Multiply/2
  Add/1 -> h_R_sp/1

== system FMS/FMS_Commander/Commander/Arm/SubMode/Return/Position Command/L1 Control ==
  p1 : Inport
  p2 : Inport  Port=2
  p3 : Inport  Port=3
  FMS_In : Inport  Port=4
  Bus Selector1 : BusSelector  OutputSignals=INS_Out.vn,INS_Out.ve
  L1 : Constant  Value=FMS_PARAM.L1  OutDataTypeStr=single
  L1 Reference WP : Subsystem
  L1_Core : Subsystem
  Mux : Mux  Inputs=2
  Saturation1 : Saturate  UpperLimit=FMS_PARAM.ACC_Y_LIM  LowerLimit=-FMS_PARAM.ACC_Y_LIM
  ay_cmd_mPs2 : Outport  VectorParamsAs1DForOutWhenUnconnected=off
  wires:
  p3/1 -> L1_Core/1(p_vehicle), L1 Reference WP/3(P3)
  p2/1 -> L1 Reference WP/2(P2)
  p1/1 -> L1 Reference WP/1(P1)
  L1/1 -> L1_Core/3(L1), L1 Reference WP/4(L1)
  L1 Reference WP/1(L1_WP) -> L1_Core/2(L1_WP)  "L1_WP"
  Mux/1 -> L1_Core/4(Vg)
  Bus Selector1/1 -> Mux/1  "<vn>"
  Bus Selector1/2 -> Mux/2  "<ve>"
  FMS_In/1 -> Bus Selector1/1
  L1_Core/1(ay_cmd_mPs2) -> Saturation1/1
  Saturation1/1 -> ay_cmd_mPs2/1

== system FMS/FMS_Commander/Commander/Arm/SubMode/Return/Position Command/WayPoints ==
  note: P1: path start point
      | P2: path end point
      | P3: vehicle point
  FMS_In : Inport
  Bus Selector : BusSelector  OutputSignals=INS_Out.x_R,INS_Out.y_R
  Bus Selector1 : BusSelector  OutputSignals=Cmd_In.sp_waypoint
  Bus Selector2 : BusSelector  OutputSignals=Cmd_In.cur_waypoint
  Mux : Mux  Inputs=2
  Reshape : Reshape  OutputDimensionality=Customize  OutputDimensions=[2,1]
  Reshape1 : Reshape  OutputDimensionality=Customize  OutputDimensions=[2,1]
  Reshape2 : Reshape  OutputDimensionality=Customize  OutputDimensions=[2,1]
  Selector : Selector  InputPortWidth=3  IndexOptions=Index vector (dialog)  Indices=[1 2]  OutputSizes=1
  Selector1 : Selector  InputPortWidth=3  IndexOptions=Index vector (dialog)  Indices=[1 2]  OutputSizes=1
  p1 : Outport  VectorParamsAs1DForOutWhenUnconnected=off
  p2 : Outport  Port=2  VectorParamsAs1DForOutWhenUnconnected=off
  p3 : Outport  Port=3  VectorParamsAs1DForOutWhenUnconnected=off
  wires:
  Reshape2/1 -> p3/1
  Reshape1/1 -> p1/1
  Reshape/1 -> p2/1
  Bus Selector/2 -> Mux/2  "<y_R>"
  Bus Selector/1 -> Mux/1  "<x_R>"
  Mux/1 -> Reshape2/1
  Bus Selector1/1 -> Selector/1  "<sp_waypoint>"
  Selector/1 -> Reshape/1
  Selector1/1 -> Reshape1/1
  Bus Selector2/1 -> Selector1/1  "<cur_waypoint>"
  FMS_In/1 -> Bus Selector2/1, Bus Selector1/1, Bus Selector/1

== system FMS/FMS_Commander/Commander/Arm/SubMode/Takeoff/Altitude Control/Target Height ==
  FMS_In : Inport
  Add : Sum
  Bus Selector : BusSelector  OutputSignals=Cmd_In.sp_waypoint,Cmd_In.cur_waypoint
  Bus Selector1 : BusSelector  OutputSignals=INS_Out.x_R,INS_Out.y_R
  Bus Selector2 : BusSelector  OutputSignals=Cmd_In.cur_waypoint,Cmd_In.sp_waypoint
  Divide : Product  Inputs=*/
  Multiply : Product
  Mux : Mux  Inputs=2
  Saturation : Saturate  UpperLimit=1  LowerLimit=0
  Selector : Selector  InputPortWidth=3  IndexOptions=Index vector (dialog)  Indices=3  OutputSizes=1
  Selector1 : Selector  InputPortWidth=3  IndexOptions=Index vector (dialog)  Indices=3  OutputSizes=1
  Selector2 : Selector  InputPortWidth=3  IndexOptions=Index vector (dialog)  Indices=[1 2]  OutputSizes=1
  Selector3 : Selector  InputPortWidth=3  IndexOptions=Index vector (dialog)  Indices=[1 2]  OutputSizes=1
  Subtract : Sum  Inputs=+-
  Sum : Sum  Inputs=|+-
  Sum1 : Sum  Inputs=-+|
  Vector Modulus : FMT_Model_Lib/Math/Vector Modulus
      settings: SourceProductName=FMT Toolbox
  Vector Modulus1 : FMT_Model_Lib/Math/Vector Modulus
      settings: SourceProductName=FMT Toolbox
  h_R_sp : Outport  VectorParamsAs1DForOutWhenUnconnected=off
  wires:
  Multiply/1 -> Add/2
  Bus Selector1/1 -> Mux/1  "<x_R>"
  Bus Selector/1 -> Selector1/1  "<sp_waypoint>"
  Vector Modulus1/1 -> Divide/2
  Sum1/1 -> Vector Modulus1/1
  Sum/1 -> Vector Modulus/1
  Selector2/1 -> Sum1/1, Sum/2
  FMS_In/1 -> Bus Selector2/1, Bus Selector1/1, Bus Selector/1
  Bus Selector2/2 -> Selector3/1  "<sp_waypoint>"
  Vector Modulus/1 -> Divide/1
  Bus Selector1/2 -> Mux/2  "<y_R>"
  Bus Selector2/1 -> Selector2/1  "<cur_waypoint>"
  Selector1/1 -> Subtract/1
  Mux/1 -> Sum/1
  Subtract/1 -> Multiply/1
  Divide/1 -> Saturation/1
  Selector3/1 -> Sum1/2
  Bus Selector/2 -> Selector/1  "<cur_waypoint>"
  Selector/1 -> Add/1, Subtract/2
  Saturation/1 -> Multiply/2
  Add/1 -> h_R_sp/1

== system FMS/FMS_Commander/Commander/Arm/SubMode/Takeoff/Position Command/L1 Control ==
  p1 : Inport
  p2 : Inport  Port=2
  p3 : Inport  Port=3
  FMS_In : Inport  Port=4
  Bus Selector1 : BusSelector  OutputSignals=INS_Out.vn,INS_Out.ve
  L1 : Constant  Value=FMS_PARAM.L1  OutDataTypeStr=single
  L1 Reference WP : Subsystem
  L1_Core : Subsystem
  Mux : Mux  Inputs=2
  Saturation1 : Saturate  UpperLimit=FMS_PARAM.ACC_Y_LIM  LowerLimit=-FMS_PARAM.ACC_Y_LIM
  ay_cmd_mPs2 : Outport  VectorParamsAs1DForOutWhenUnconnected=off
  wires:
  p3/1 -> L1_Core/1(p_vehicle), L1 Reference WP/3(P3)
  p2/1 -> L1 Reference WP/2(P2)
  p1/1 -> L1 Reference WP/1(P1)
  L1/1 -> L1_Core/3(L1), L1 Reference WP/4(L1)
  L1 Reference WP/1(L1_WP) -> L1_Core/2(L1_WP)  "L1_WP"
  Mux/1 -> L1_Core/4(Vg)
  Bus Selector1/1 -> Mux/1  "<vn>"
  Bus Selector1/2 -> Mux/2  "<ve>"
  FMS_In/1 -> Bus Selector1/1
  L1_Core/1(ay_cmd_mPs2) -> Saturation1/1
  Saturation1/1 -> ay_cmd_mPs2/1

== system FMS/FMS_Commander/Commander/Arm/SubMode/Takeoff/Position Command/WayPoints ==
  note: P1: path start point
      | P2: path end point
      | P3: vehicle point
  FMS_In : Inport
  Bus Selector : BusSelector  OutputSignals=INS_Out.x_R,INS_Out.y_R
  Bus Selector1 : BusSelector  OutputSignals=Cmd_In.sp_waypoint
  Bus Selector2 : BusSelector  OutputSignals=Cmd_In.cur_waypoint
  Mux : Mux  Inputs=2
  Reshape : Reshape  OutputDimensionality=Customize  OutputDimensions=[2,1]
  Reshape1 : Reshape  OutputDimensionality=Customize  OutputDimensions=[2,1]
  Reshape2 : Reshape  OutputDimensionality=Customize  OutputDimensions=[2,1]
  Selector : Selector  InputPortWidth=3  IndexOptions=Index vector (dialog)  Indices=[1 2]  OutputSizes=1
  Selector1 : Selector  InputPortWidth=3  IndexOptions=Index vector (dialog)  Indices=[1 2]  OutputSizes=1
  p1 : Outport  VectorParamsAs1DForOutWhenUnconnected=off
  p2 : Outport  Port=2  VectorParamsAs1DForOutWhenUnconnected=off
  p3 : Outport  Port=3  VectorParamsAs1DForOutWhenUnconnected=off
  wires:
  Reshape2/1 -> p3/1
  Reshape1/1 -> p1/1
  Reshape/1 -> p2/1
  Bus Selector/2 -> Mux/2  "<y_R>"
  Bus Selector/1 -> Mux/1  "<x_R>"
  Mux/1 -> Reshape2/1
  FMS_In/1 -> Bus Selector2/1, Bus Selector1/1, Bus Selector/1
  Bus Selector1/1 -> Selector/1  "<sp_waypoint>"
  Selector/1 -> Reshape/1
  Bus Selector2/1 -> Selector1/1  "<cur_waypoint>"
  Selector1/1 -> Reshape1/1

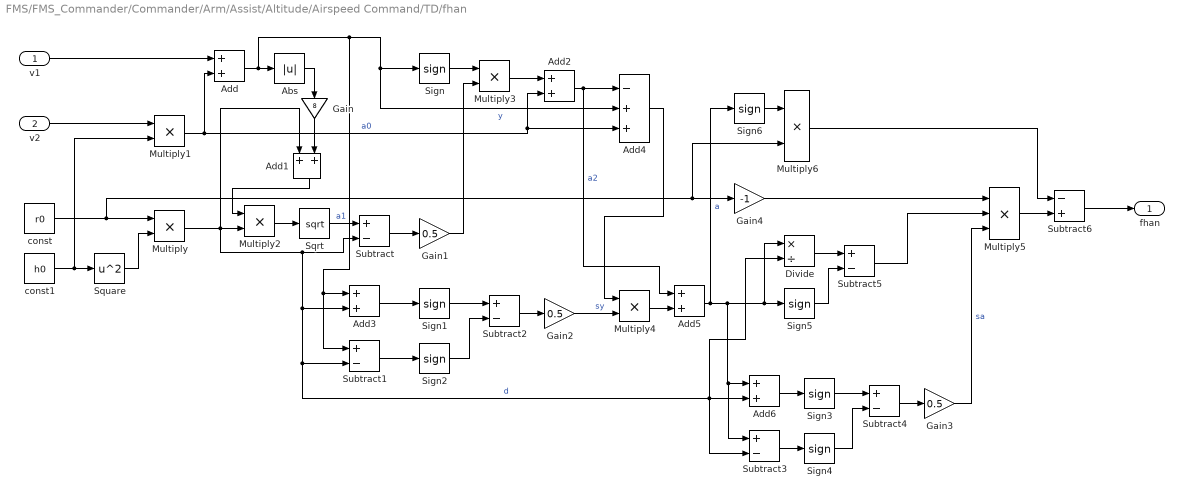
== system FMS/FMS_Commander/Commander/Arm/Assist/Altitude/Airspeed Command/TD/fhan  ==
  v1 : Inport
  v2 : Inport  Port=2
  Abs : Abs
  Add{,1..3,5..6} (6 alike) : Sum  OutDataTypeStr=Inherit: Same as first input
  Add4 : Sum  Inputs=-++
  Divide : Product  Inputs=*/
  Gain : Gain  Gain=8
  Gain1 : Gain  Gain=0.5  OutDataTypeStr=Inherit: Same as input
  Gain2 : Gain  Gain=0.5  OutDataTypeStr=Inherit: Same as input
  Gain3 : Gain  Gain=0.5  OutDataTypeStr=Inherit: Same as input
  Gain4 : Gain  Gain=-1  OutDataTypeStr=Inherit: Same as input
  Multiply{,1..3} (4 alike) : Product  OutDataTypeStr=Inherit: Same as first input
  Multiply4 : Product  OutDataTypeStr=single
  Multiply5 : Product  Inputs=3
  Multiply6 : Product  OutDataTypeStr=single
  Sign{,1..6} (7 alike) : Signum
  Sqrt : Sqrt  SaturateOnIntegerOverflow=on
  Square : Math  Operator=square  SaturateOnIntegerOverflow=on
  Subtract{,1..5} (6 alike) : Sum  Inputs=+-  OutDataTypeStr=Inherit: Same as first input
  Subtract6 : Sum  Inputs=-+  OutDataTypeStr=Inherit: Same as first input
  const : Constant  Value=r0  OutDataTypeStr=single
  const1 : Constant  Value=h0  OutDataTypeStr=single
  fhan : Outport  VectorParamsAs1DForOutWhenUnconnected=off
  wires:
  Sign1/1 -> Subtract2/1
  Multiply2/1 -> Sqrt/1
  Square/1 -> Multiply/2
  Gain1/1 -> Multiply3/2
  Multiply6/1 -> Subtract6/1
  Multiply/1 -> Multiply2/2, Add1/1, Add3/2, Subtract1/2, Add6/2, Subtract3/2, Divide/2, Subtract/2  "d"
  Add6/1 -> Sign3/1
  Sign3/1 -> Subtract4/1
  Sign6/1 -> Multiply6/1
  Multiply5/1 -> Subtract6/2
  Gain4/1 -> Multiply5/1
  Subtract4/1 -> Gain3/1
  Add2/1 -> Add5/1, Add4/1  "a2"
  Subtract2/1 -> Gain2/1
  Add/1 -> Abs/1, Sign/1, Add4/2, Add3/1, Subtract1/1  "y"
  Multiply1/1 -> Add/2, Add2/2, Add4/3  "a0"
  Add5/1 -> Add6/1, Subtract3/1, Divide/1, Sign5/1, Sign6/1  "a"
  const1/1 -> Square/1, Multiply1/2
  Multiply4/1 -> Add5/2
  Subtract5/1 -> Multiply5/2
  Add3/1 -> Sign1/1
  const/1 -> Multiply/1, Gain4/1, Multiply6/2
  Gain/1 -> Add1/2
  Multiply3/1 -> Add2/1
  Divide/1 -> Subtract5/1
  Subtract1/1 -> Sign2/1
  Add1/1 -> Multiply2/1
  Subtract3/1 -> Sign4/1
  Sqrt/1 -> Subtract/1  "a1"
  Sign5/1 -> Subtract5/2
  Add4/1 -> Multiply4/1
  Abs/1 -> Gain/1
  Sign4/1 -> Subtract4/2
  Sign2/1 -> Subtract2/2
  Subtract6/1 -> fhan/1
  Subtract/1 -> Gain1/1
  Gain3/1 -> Multiply5/3  "sa"
  v2/1 -> Multiply1/1
  Gain2/1 -> Multiply4/2  "sy"
  Sign/1 -> Multiply3/1
  v1/1 -> Add/1

== system FMS/FMS_Commander/Commander/Arm/Assist/Altitude/Altitude Command/Controller/Brake Control ==
  Action Port : ActionPort  InitializeStates=reset
  Brake Speed : Constant  Value=0  VectorParams1D=off  OutDataTypeStr=single
  psi_rate_cmd_radPs : Outport  VectorParamsAs1DForOutWhenUnconnected=off
  wires:
  Brake Speed/1 -> psi_rate_cmd_radPs/1

== system FMS/FMS_Commander/Commander/Arm/Assist/Altitude/Altitude Command/Controller/Hold Control ==
  FMS_In : Inport
  Action Port : ActionPort  InitializeStates=reset
  Bus_Selection : Subsystem
  Delay : Delay  DelayLength=1  InitialConditionSource=Input port
      settings: InputPortMap=u0,p4
  Gain2 : Gain  Gain=FMS_PARAM.Z_P  OutDataTypeStr=single
  Sum : Sum  Inputs=-+|
  w_cmd_mPs : Outport  VectorParamsAs1DForOutWhenUnconnected=off
  wires:
  FMS_In/1 -> Bus_Selection/1(FMS_In)
  Delay/1 -> Sum/2, Delay/1  "z_cmd_R"
  Sum/1 -> Gain2/1  "z_err_R"
  Bus_Selection/1(z_R_m) -> Delay/2, Sum/1  "z_est_R"
  Gain2/1 -> w_cmd_mPs/1

== system FMS/FMS_Commander/Commander/Arm/Assist/Altitude/Altitude Command/Controller/Move Control ==
  FMS_In : Inport
  Action Port : ActionPort  InitializeStates=reset
  Bus Selector : BusSelector  OutputSignals=Pilot_Cmd.stick_pitch
  DeadZone : Subsystem  mask{th=FMS_PARAM.PITCH_DZ}
      mask prompts: th "Threshold"
      mask Display: disp('Dead Zone')
  Gain1 : Gain  Gain=FMS_PARAM.VEL_Z_LIM  OutDataTypeStr=single
  TD1 : Subsystem  Commented=on
  w_cmd_mPs : Outport  VectorParamsAs1DForOutWhenUnconnected=off
  wires:
  FMS_In/1 -> Bus Selector/1
  Bus Selector/1 -> DeadZone/1(u)  "<stick_pitch>"
  DeadZone/1(y) -> Gain1/1
  Gain1/1 -> w_cmd_mPs/1

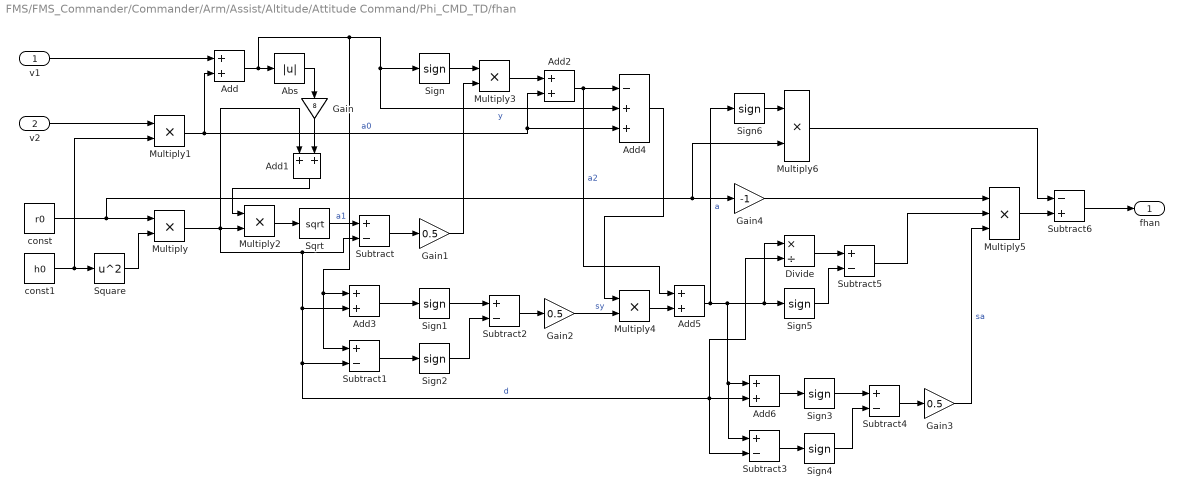
== system FMS/FMS_Commander/Commander/Arm/Assist/Altitude/Attitude Command/Phi_CMD_TD/fhan  ==
  v1 : Inport
  v2 : Inport  Port=2
  Abs : Abs
  Add{,1..3,5..6} (6 alike) : Sum  OutDataTypeStr=Inherit: Same as first input
  Add4 : Sum  Inputs=-++
  Divide : Product  Inputs=*/
  Gain : Gain  Gain=8
  Gain1 : Gain  Gain=0.5  OutDataTypeStr=Inherit: Same as input
  Gain2 : Gain  Gain=0.5  OutDataTypeStr=Inherit: Same as input
  Gain3 : Gain  Gain=0.5  OutDataTypeStr=Inherit: Same as input
  Gain4 : Gain  Gain=-1  OutDataTypeStr=Inherit: Same as input
  Multiply{,1..3} (4 alike) : Product  OutDataTypeStr=Inherit: Same as first input
  Multiply4 : Product  OutDataTypeStr=single
  Multiply5 : Product  Inputs=3
  Multiply6 : Product  OutDataTypeStr=single
  Sign{,1..6} (7 alike) : Signum
  Sqrt : Sqrt  SaturateOnIntegerOverflow=on
  Square : Math  Operator=square  SaturateOnIntegerOverflow=on
  Subtract{,1..5} (6 alike) : Sum  Inputs=+-  OutDataTypeStr=Inherit: Same as first input
  Subtract6 : Sum  Inputs=-+  OutDataTypeStr=Inherit: Same as first input
  const : Constant  Value=r0  OutDataTypeStr=single
  const1 : Constant  Value=h0  OutDataTypeStr=single
  fhan : Outport  VectorParamsAs1DForOutWhenUnconnected=off
  wires:
  v1/1 -> Add/1
  Sign/1 -> Multiply3/1
  Gain2/1 -> Multiply4/2  "sy"
  v2/1 -> Multiply1/1
  Gain3/1 -> Multiply5/3  "sa"
  Subtract/1 -> Gain1/1
  Subtract6/1 -> fhan/1
  Sign2/1 -> Subtract2/2
  Sign4/1 -> Subtract4/2
  Abs/1 -> Gain/1
  Add4/1 -> Multiply4/1
  Sign5/1 -> Subtract5/2
  Sqrt/1 -> Subtract/1  "a1"
  Subtract3/1 -> Sign4/1
  Add1/1 -> Multiply2/1
  Subtract1/1 -> Sign2/1
  Divide/1 -> Subtract5/1
  Multiply3/1 -> Add2/1
  Gain/1 -> Add1/2
  const/1 -> Multiply6/2, Gain4/1, Multiply/1
  Add3/1 -> Sign1/1
  Subtract5/1 -> Multiply5/2
  Multiply4/1 -> Add5/2
  const1/1 -> Multiply1/2, Square/1
  Add5/1 -> Sign6/1, Sign5/1, Divide/1, Subtract3/1, Add6/1  "a"
  Multiply1/1 -> Add4/3, Add2/2, Add/2  "a0"
  Add/1 -> Subtract1/1, Add3/1, Add4/2, Sign/1, Abs/1  "y"
  Subtract2/1 -> Gain2/1
  Add2/1 -> Add4/1, Add5/1  "a2"
  Subtract4/1 -> Gain3/1
  Gain4/1 -> Multiply5/1
  Multiply5/1 -> Subtract6/2
  Sign6/1 -> Multiply6/1
  Sign3/1 -> Subtract4/1
  Add6/1 -> Sign3/1
  Multiply/1 -> Subtract/2, Divide/2, Subtract3/2, Add6/2, Subtract1/2, Add3/2, Add1/1, Multiply2/2  "d"
  Multiply6/1 -> Subtract6/1
  Gain1/1 -> Multiply3/2
  Square/1 -> Multiply/2
  Multiply2/1 -> Sqrt/1
  Sign1/1 -> Subtract2/1

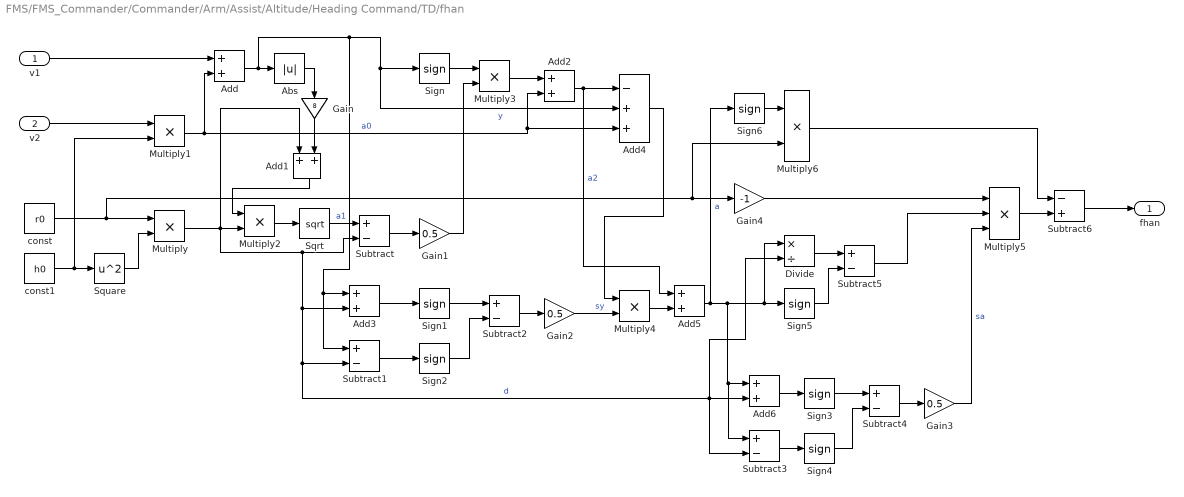
== system FMS/FMS_Commander/Commander/Arm/Assist/Altitude/Heading Command/TD/fhan  ==
  v1 : Inport
  v2 : Inport  Port=2
  Abs : Abs
  Add{,1..3,5..6} (6 alike) : Sum  OutDataTypeStr=Inherit: Same as first input
  Add4 : Sum  Inputs=-++
  Divide : Product  Inputs=*/
  Gain : Gain  Gain=8
  Gain1 : Gain  Gain=0.5  OutDataTypeStr=Inherit: Same as input
  Gain2 : Gain  Gain=0.5  OutDataTypeStr=Inherit: Same as input
  Gain3 : Gain  Gain=0.5  OutDataTypeStr=Inherit: Same as input
  Gain4 : Gain  Gain=-1  OutDataTypeStr=Inherit: Same as input
  Multiply{,1..3} (4 alike) : Product  OutDataTypeStr=Inherit: Same as first input
  Multiply4 : Product  OutDataTypeStr=single
  Multiply5 : Product  Inputs=3
  Multiply6 : Product  OutDataTypeStr=single
  Sign{,1..6} (7 alike) : Signum
  Sqrt : Sqrt  SaturateOnIntegerOverflow=on
  Square : Math  Operator=square  SaturateOnIntegerOverflow=on
  Subtract{,1..5} (6 alike) : Sum  Inputs=+-  OutDataTypeStr=Inherit: Same as first input
  Subtract6 : Sum  Inputs=-+  OutDataTypeStr=Inherit: Same as first input
  const : Constant  Value=r0  OutDataTypeStr=single
  const1 : Constant  Value=h0  OutDataTypeStr=single
  fhan : Outport  VectorParamsAs1DForOutWhenUnconnected=off
  wires:
  v1/1 -> Add/1
  Sign/1 -> Multiply3/1
  Gain2/1 -> Multiply4/2  "sy"
  v2/1 -> Multiply1/1
  Gain3/1 -> Multiply5/3  "sa"
  Subtract/1 -> Gain1/1
  Subtract6/1 -> fhan/1
  Sign2/1 -> Subtract2/2
  Sign4/1 -> Subtract4/2
  Abs/1 -> Gain/1
  Add4/1 -> Multiply4/1
  Sign5/1 -> Subtract5/2
  Sqrt/1 -> Subtract/1  "a1"
  Subtract3/1 -> Sign4/1
  Add1/1 -> Multiply2/1
  Subtract1/1 -> Sign2/1
  Divide/1 -> Subtract5/1
  Multiply3/1 -> Add2/1
  Gain/1 -> Add1/2
  const/1 -> Multiply6/2, Gain4/1, Multiply/1
  Add3/1 -> Sign1/1
  Subtract5/1 -> Multiply5/2
  Multiply4/1 -> Add5/2
  const1/1 -> Multiply1/2, Square/1
  Add5/1 -> Sign6/1, Sign5/1, Divide/1, Subtract3/1, Add6/1  "a"
  Multiply1/1 -> Add4/3, Add2/2, Add/2  "a0"
  Add/1 -> Subtract1/1, Add3/1, Add4/2, Sign/1, Abs/1  "y"
  Subtract2/1 -> Gain2/1
  Add2/1 -> Add4/1, Add5/1  "a2"
  Subtract4/1 -> Gain3/1
  Gain4/1 -> Multiply5/1
  Multiply5/1 -> Subtract6/2
  Sign6/1 -> Multiply6/1
  Sign3/1 -> Subtract4/1
  Add6/1 -> Sign3/1
  Multiply/1 -> Subtract/2, Divide/2, Subtract3/2, Add6/2, Subtract1/2, Add3/2, Add1/1, Multiply2/2  "d"
  Multiply6/1 -> Subtract6/1
  Gain1/1 -> Multiply3/2
  Square/1 -> Multiply/2
  Multiply2/1 -> Sqrt/1
  Sign1/1 -> Subtract2/1

== system FMS/FMS_Commander/Commander/Arm/Assist/Position/Altitude Command/Controller/Brake Control ==
  Action Port : ActionPort  InitializeStates=reset
  Brake Speed : Constant  Value=0  VectorParams1D=off  OutDataTypeStr=single
  psi_rate_cmd_radPs : Outport  VectorParamsAs1DForOutWhenUnconnected=off
  wires:
  Brake Speed/1 -> psi_rate_cmd_radPs/1

== system FMS/FMS_Commander/Commander/Arm/Assist/Position/Altitude Command/Controller/Hold Control ==
  FMS_In : Inport
  Action Port : ActionPort  InitializeStates=reset
  Bus_Selection : Subsystem
  Delay : Delay  DelayLength=1  InitialConditionSource=Input port
      settings: InputPortMap=u0,p4
  Gain2 : Gain  Gain=FMS_PARAM.Z_P  OutDataTypeStr=single
  Sum : Sum  Inputs=-+|
  w_cmd_mPs : Outport  VectorParamsAs1DForOutWhenUnconnected=off
  wires:
  FMS_In/1 -> Bus_Selection/1(FMS_In)
  Delay/1 -> Sum/2, Delay/1  "z_cmd_R"
  Sum/1 -> Gain2/1  "z_err_R"
  Bus_Selection/1(z_R_m) -> Delay/2, Sum/1  "z_est_R"
  Gain2/1 -> w_cmd_mPs/1

== system FMS/FMS_Commander/Commander/Arm/Assist/Position/Altitude Command/Controller/Move Control ==
  FMS_In : Inport
  Action Port : ActionPort  InitializeStates=reset
  Bus Selector : BusSelector  OutputSignals=Pilot_Cmd.stick_pitch
  DeadZone : Subsystem  mask{th=FMS_PARAM.PITCH_DZ}
      mask prompts: th "Threshold"
      mask Display: disp('Dead Zone')
  Gain1 : Gain  Gain=FMS_PARAM.VEL_Z_LIM  OutDataTypeStr=single
  TD1 : Subsystem  Commented=on
  w_cmd_mPs : Outport  VectorParamsAs1DForOutWhenUnconnected=off
  wires:
  Gain1/1 -> w_cmd_mPs/1
  FMS_In/1 -> Bus Selector/1
  Bus Selector/1 -> DeadZone/1(u)  "<stick_pitch>"
  DeadZone/1(y) -> Gain1/1
